simulink model "sim_rbf3"  (R2023a)
settings: Solver=VariableStepAuto  StartTime=0.0  StopTime=10  RelTol=1e-3
settings Model: Creator=ACCENT  LastModifiedBy=ACCENT

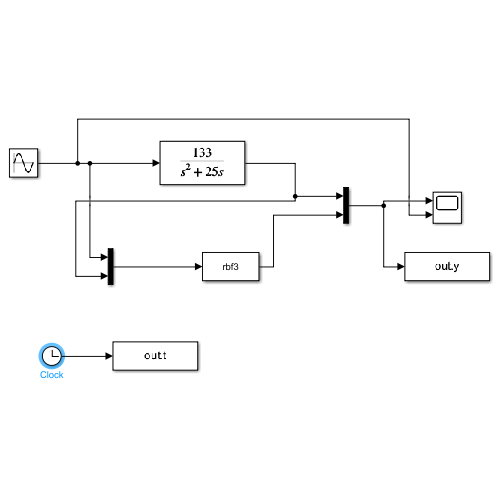
[thumbnail: Simulink's stored preview of the top-level diagram]
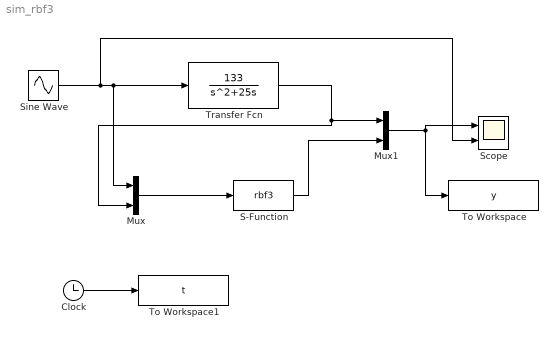
== system sim_rbf3 ==
  Clock : Clock
  Mux : Mux  Inputs=2
  Mux1 : Mux  Inputs=2
  S-Function : S-Function  FunctionName=rbf3  SFunctionDeploymentMode=off  EnableBusSupport=off
  Scope : Scope  NumInputPorts=2
  Sine Wave : Sin  SampleTime=0
  To Workspace : ToWorkspace  VariableName=y  SampleTime=-1
  To Workspace1 : ToWorkspace  VariableName=t  SampleTime=-1
  Transfer Fcn : TransferFcn  Numerator=133  Denominator=[1 25 0]
  wires:
  Clock/1 -> To Workspace1/1
  Sine Wave/1 -> Scope/2, Transfer Fcn/1, Mux/1
  Mux/1 -> S-Function/1
  S-Function/1 -> Mux1/2
  Mux1/1 -> To Workspace/1, Scope/1
  Transfer Fcn/1 -> Mux/2, Mux1/1
